simulink model "Sub_SC_G_based_221004"  (R2022b)
settings: Solver=VariableStepAuto  StartTime=0.0  StopTime=SimTime  RelTol=1e-3
undefined symbols (not defined in the file or in its folder): R_bal, SC_PreChgTime, SC_rc, SC_rv
libraries: spsCurrentMeasurementLib x14, spsSeriesRLCBranchLib x13, spsSupercapacitorLib x12, spsIdealSwitchLib x3, spsDCVoltageSourceLib x2, spsVariableResistorLib x2, spsVoltageMeasurementLib x1, sps_lib x1
settings Model: Creator=xuupp  LastModifiedBy=xuupp

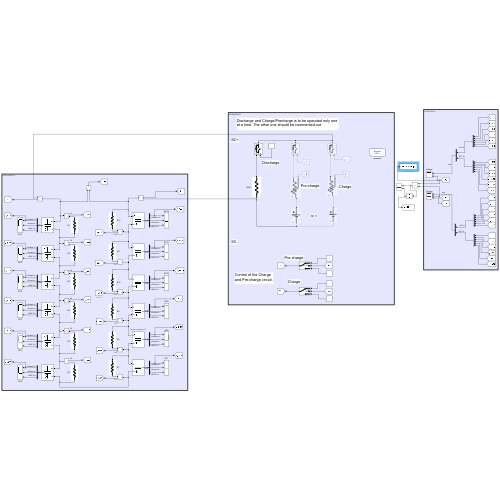
[thumbnail: Simulink's stored preview of the top-level diagram]
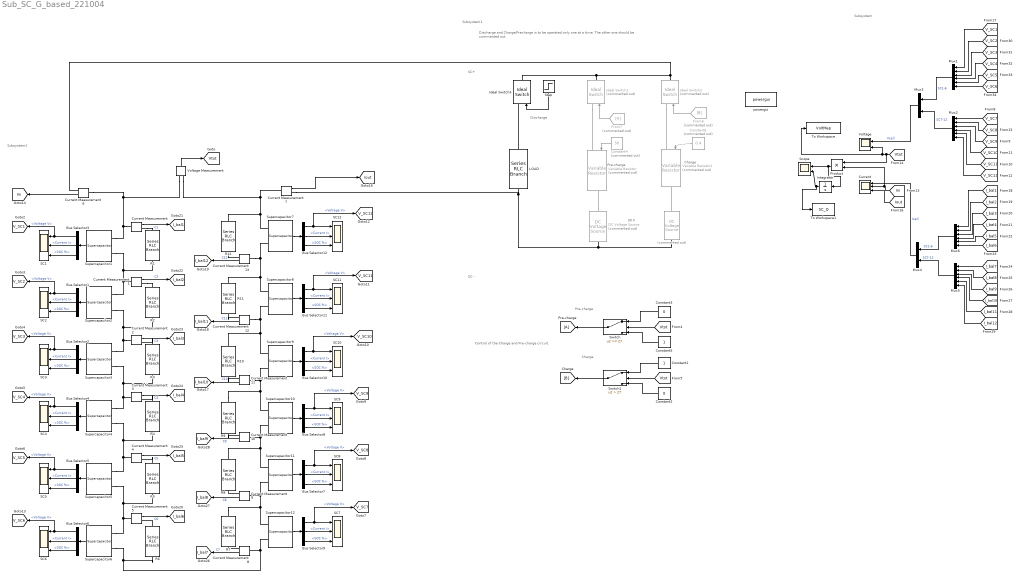
== system Sub_SC_G_based_221004 ==
  note: Pre-charge
  note: Subsystem2
  note: Control of the Charge and Pre-charge circuit.
  note: Subsystem
  note: 30 V
  note: Subsystem1
  note: SC -
  note: Charge
  note: Pre-charge
  note: SC+
  note: Discharge and Charge/Precharge is to be operated only one at a time. The other one should be commented out.
  note: Charge
  note: Discharge
  " " : spsDCVoltageSourceLib/DC Voltage Source  Commented=on  Amplitude=30  Measurements=None
  Bus Selector{1..12} (12 alike) : BusSelector  OutputSignals=Voltage V,Current I,SOC %
  Constant1 : Constant
  Constant2 : Constant  Value=0
  Constant3 : Constant  Value=0
  Constant4 : Constant  Commented=on  Value=30
  Constant5 : Constant
  Constant6 : Constant  Commented=on  Value=0.4
  Current : Scope  NumInputPorts=3
  Current Measurement{,1..13} (14 alike) : spsCurrentMeasurementLib/Current Measurement  PhasorSimulation=off  OutputType=Complex  PSBequivalent=0
  DC Voltage Source : spsDCVoltageSourceLib/DC Voltage Source  Commented=on  Amplitude=30  Measurements=None
  From6 : From  Commented=on  GotoTag=B
  From7 : From  Commented=on
  Ideal Switch1 : spsIdealSwitchLib/Ideal Switch  Commented=on  Ron=0.00001  Lon=0  IC=0  Rs=1e5  Cs=inf  Measurements=off
  Ideal Switch2 : spsIdealSwitchLib/Ideal Switch  Commented=on  Ron=0.00001  Lon=0  IC=0  Rs=1e5  Cs=inf  Measurements=off
  Ideal Switch3 : spsIdealSwitchLib/Ideal Switch  Ron=0.00001  Lon=0  IC=0  Rs=1e5  Cs=inf  Measurements=off
  Integrator : Integrator
  LOAD : spsSeriesRLCBranchLib/Series RLC Branch  LConnTagsString=__new0  RConnTagsString=__new0  BranchType=R  Resistance=10  Inductance=1e-3  SetiL0=off  InitialCurrent=0  Capacitance=1e-5  Setx0=on  InitialVoltage=0  Measurements=Branch voltage and current
  Mux{1..2,5..6} (4 alike) : Mux  Inputs=6
  Mux3 : Mux  Inputs=2
  Mux4 : Mux  Inputs=2
  Pre-charge : Goto
  Product : Product
  R{1..12} (12 alike) : spsSeriesRLCBranchLib/Series RLC Branch  LConnTagsString=__new0  RConnTagsString=__new0  BranchType=R  Resistance=R_bal  Inductance=1e-3  SetiL0=off  InitialCurrent=0  Capacitance=54.3e-6  Setx0=on  InitialVoltage=160  Measurements=None
  SC{1..12} (12 alike) : Scope  NumInputPorts=3
  Scope : Scope  NumInputPorts=2
  Step : Step  Time=SC_PreChgTime  SampleTime=0
  Supercapacitor{1..12} (12 alike) : spsSupercapacitorLib/Supercapacitor  C=SC_rc  Rdc=8.9e-3  Voltage=SC_rv  Ns=1  Np=1  Vinit=SC_iv  Temp=25  PresetModel=off  EstParam=off  Nc=1  r=1e-9  epsilon=6.0208e-10  Ich=10  Vstern="[0.161  2.7  7.8]"  Self_dis=on  Ioc=10  Vself="[48  47.8  47.06  44.65]"  demandeplot=off  I="[10  20 100  500]"  Units=sec  Vmax=0  If=0  deltaV=0  alpha=0  sec=0
      settings: LibrarySourceBlock=sps_lib/Sources/Supercapacitor
  Switch : Switch  Threshold=27  SaturateOnIntegerOverflow=off  InputSameDT=off
  Switch1 : Switch  Criteria=u2 > Threshold  Threshold=27  SaturateOnIntegerOverflow=off  InputSameDT=off
  To Workspace : ToWorkspace  VariableName=VoltMap  SaveFormat=Timeseries  SampleTime=-1
  To Workspace1 : ToWorkspace  VariableName=SC_Q  SaveFormat=Structure With Time  SampleTime=-1
  Variable Resistor : spsVariableResistorLib/Variable Resistor  Commented=on  Rabsmin=1e-3
      settings: LibrarySourceBlock=sps_lib/Passives/Variable Resistor
  Variable Resistor1 : spsVariableResistorLib/Variable Resistor  Commented=on  Rabsmin=1e-3
      settings: LibrarySourceBlock=sps_lib/Passives/Variable Resistor
  Voltage : Scope  NumInputPorts=2
  Voltage Measurement : spsVoltageMeasurementLib/Voltage Measurement  PhasorSimulation=off  OutputType=Complex  PSBequivalent=0
  powergui : sps_lib/powergui  Priority=1  SimulationMode=Discrete  SampleTime=0.01  frequency=60  Iterations=50  frequencyindice=0  Pbase=100e6  ErrMax=1e-4  UnitsV=kV  UnitsW=MW  buscounter=0  FunctionMessages=off  echomessages=off  EnableUseOfTLC=off  CurrentSourceSwitches=off  DisableSnubberDevices=off  DisableRonSwitches=off  DisableVfSwitches=off  DisplayEquations=off  AutomaticDiscreteSolvers=off  SolverType=Tustin/Backward Euler (TBE)  Interpol=off  ExternalGateDelay=off  methode=off  Ts=100  x0status=blocks  SPID=on  SwTol=0  HookPort=off  NonlinearTolerance=1e-4  nMaxIteration=100  ContinueOnMaxIteration=off  RestoreLinks=warning  ResistiveCurrentMeasurement=off  Frange=[0:2:500]  Ylog=off  Xlog=on  ShowGrid=off  save=off  variable=ZData  structure=0  ZoomFFT=off  StartTime=0.0  cycles=1  DisplayStyle=1  fundamental=60  FreqAxis=off  MaxFrequency=1000  frequencyindicesteady=1  RmsSteady=1  display=off
  tag scope: I_bal10=global, I_bal11=global, I_bal12=global, I_bal1=global, I_bal2=global, I_bal3=global, I_bal4=global, I_bal5=global, I_bal6=global, I_bal7=global, I_bal8=global, I_bal9=global, Iin=global, Iout=global, V_SC10=global, V_SC11=global, V_SC12=global, V_SC1=global, V_SC2=global, V_SC3=global, V_SC4=global, V_SC5=global, V_SC6=global, V_SC7=global, V_SC8=global, V_SC9=global, Vtot=global
  wires:
  Supercapacitor4/1 -> Bus Selector4/1
  Current Measurement12/1 -> [I_bal11]  "C11"
  Bus Selector12/3 -> SC12/3  "<SOC %>"
  [I_bal7] -> Mux5/1
  Bus Selector11/2 -> SC11/2  "<Current I>"
  Supercapacitor3/1 -> Bus Selector2/1
  Bus Selector2/3 -> SC3/3  "<SOC %>"
  Current Measurement11/1 -> [I_bal10]  "C10"
  Bus Selector1/2 -> SC2/2  "<Current I>"
  From7/1 -> Ideal Switch1/1
  Constant3/1 -> Switch/1
  Bus Selector3/1 -> [V_SC1], SC1/1  "<Voltage V>"
  Current Measurement8/1 -> [I_bal7]  "C7"
  Bus Selector1/3 -> SC2/3  "<SOC %>"
  Current Measurement1/1 -> [I_bal2]  "C2"
  Current Measurement5/1 -> [I_bal6]  "C6"
  Bus Selector5/1 -> [V_SC5], SC5/1  "<Voltage V>"
  Bus Selector10/2 -> SC10/2  "<Current I>"
  Bus Selector7/3 -> SC8/3  "<SOC %>"
  Bus Selector11/1 -> [V_SC11], SC11/1  "<Voltage V>"
  Bus Selector2/2 -> SC3/2  "<Current I>"
  Bus Selector4/3 -> SC4/3  "<SOC %>"
  Supercapacitor2/1 -> Bus Selector1/1
  Current Measurement/1 -> [I_bal1]  "C1"
  Bus Selector1/1 -> [V_SC2], SC2/1  "<Voltage V>"
  Bus Selector8/2 -> SC9/2  "<Current I>"
  Supercapacitor8/1 -> Bus Selector11/1
  Current Measurement2/1 -> [I_bal3]  "C3"
  Bus Selector8/3 -> SC9/3  "<SOC %>"
  Current Measurement6/1 -> [Iin]
  Bus Selector5/3 -> SC5/3  "<SOC %>"
  Bus Selector2/1 -> [V_SC3], SC3/1  "<Voltage V>"
  Bus Selector6/2 -> SC6/2  "<Current I>"
  Supercapacitor12/1 -> Bus Selector9/1
  Supercapacitor5/1 -> Bus Selector5/1
  Bus Selector12/2 -> SC12/2  "<Current I>"
  Supercapacitor7/1 -> Bus Selector12/1
  Bus Selector7/2 -> SC8/2  "<Current I>"
  Constant5/1 -> Switch/3
  Constant1/1 -> Switch1/1
  From6/1 -> Ideal Switch2/1
  [Vtot] -> Switch/2
  [Vtot] -> Switch1/2
  Switch/1 -> Pre-charge/1
  Step/1 -> Ideal Switch3/1
  Current Measurement9/1 -> [I_bal8]  "C8"
  Voltage Measurement/1 -> [Vtot]
  Current Measurement3/1 -> [I_bal4]  "C4"
  Constant4/1 -> Variable Resistor/1
  [V_SC4] -> Mux1/4
  [I_bal10] -> Mux5/4
  [V_SC12] -> Mux2/6
  [V_SC3] -> Mux1/3
  Bus Selector7/1 -> [V_SC8], SC8/1  "<Voltage V>"
  [I_bal3] -> Mux6/3
  [Vtot] -> Product/1, To Workspace/1, Voltage/2
  Bus Selector3/3 -> SC1/3  "<SOC %>"
  Supercapacitor6/1 -> Bus Selector6/1
  Bus Selector12/1 -> [V_SC12], SC12/1  "<Voltage V>"
  Bus Selector6/3 -> SC6/3  "<SOC %>"
  Bus Selector4/2 -> SC4/2  "<Current I>"
  Current Measurement10/1 -> [I_bal9]  "C9"
  Bus Selector6/1 -> [V_SC6], SC6/1  "<Voltage V>"
  [I_bal11] -> Mux5/5
  [V_SC8] -> Mux2/2
  [I_bal12] -> Mux5/6
  [I_bal2] -> Mux6/2
  [V_SC7] -> Mux2/1
  Constant6/1 -> Variable Resistor1/1
  Mux1/1 -> Mux3/1  "SC1-6"
  [I_bal9] -> Mux5/3
  Bus Selector10/3 -> SC10/3  "<SOC %>"
  Mux3/1 -> Voltage/1  "Vcell"
  [V_SC1] -> Mux1/1
  Bus Selector9/2 -> SC7/2  "<Current I>"
  Bus Selector9/1 -> [V_SC7], SC7/1  "<Voltage V>"
  Switch1/1 -> [B]
  Supercapacitor11/1 -> Bus Selector7/1
  [Iout] -> Current/3
  Bus Selector10/1 -> [V_SC10], SC10/1  "<Voltage V>"
  [V_SC9] -> Mux2/3
  Bus Selector11/3 -> SC11/3  "<SOC %>"
  Supercapacitor10/1 -> Bus Selector8/1
  Bus Selector9/3 -> SC7/3  "<SOC %>"
  Bus Selector8/1 -> [V_SC9], SC9/1  "<Voltage V>"
  [I_bal5] -> Mux6/5
  [I_bal8] -> Mux5/2
  Supercapacitor9/1 -> Bus Selector10/1
  [V_SC10] -> Mux2/4
  [I_bal4] -> Mux6/4
  Mux5/1 -> Mux4/2  "SC7-12"
  Bus Selector4/1 -> [V_SC4], SC4/1  "<Voltage V>"
  [V_SC2] -> Mux1/2
  Current Measurement7/1 -> [Iout]
  Bus Selector5/2 -> SC5/2  "<Current I>"
  Constant2/1 -> Switch1/3
  [V_SC5] -> Mux1/5
  [Iin] -> Product/2, Current/2
  Supercapacitor1/1 -> Bus Selector3/1
  Bus Selector3/2 -> SC1/2  "<Current I>"
  Current Measurement13/1 -> [I_bal12]  "C12"
  Mux4/1 -> Current/1  "Icell"
  Mux6/1 -> Mux4/1  "SC1-6"
  [I_bal1] -> Mux6/1
  [I_bal6] -> Mux6/6
  [V_SC11] -> Mux2/5
  Current Measurement4/1 -> [I_bal5]  "C5"
  [V_SC6] -> Mux1/6
  Mux2/1 -> Mux3/2  "SC7-12"
  Product/1 -> Integrator/1, Scope/1
  Integrator/1 -> To Workspace1/1, Scope/2
  connections:
  R6/RConn1 -- Supercapacitor6/LConn2 -- Supercapacitor12/LConn1 -- Current Measurement8/LConn1
  Current Measurement13/LConn1 -- Supercapacitor7/LConn1 -- Supercapacitor8/LConn2 -- R11/RConn1
  Current Measurement/LConn1 -- Supercapacitor1/LConn1 -- Voltage Measurement/LConn1 -- Current Measurement6/LConn1
  Current Measurement12/LConn1 -- Supercapacitor8/LConn1 -- Supercapacitor9/LConn2 -- R10/RConn1
  Current Measurement2/LConn1 -- Supercapacitor3/LConn1 -- Supercapacitor2/LConn2 -- R2/RConn1
  R9/RConn1 -- Supercapacitor10/LConn2 -- Supercapacitor9/LConn1 -- Current Measurement11/LConn1
  Current Measurement10/LConn1 -- Supercapacitor10/LConn1 -- Supercapacitor11/LConn2 -- R8/RConn1
  R1/RConn1 -- Supercapacitor1/LConn2 -- Supercapacitor2/LConn1 -- Current Measurement1/LConn1
  Ideal Switch3/RConn1 -- Ideal Switch1/RConn1 -- Ideal Switch2/RConn1 -- Current Measurement6/RConn1
  R4/RConn1 -- Supercapacitor4/LConn2 -- Supercapacitor5/LConn1 -- Current Measurement4/LConn1
  R5/RConn1 -- Supercapacitor5/LConn2 -- Supercapacitor6/LConn1 -- Current Measurement5/LConn1
  Voltage Measurement/LConn2 -- Supercapacitor7/LConn2 -- R12/RConn1 -- Current Measurement7/LConn1
  LOAD/RConn1 -- " "/LConn1 -- DC Voltage Source/LConn1 -- Current Measurement7/RConn1
  R7/RConn1 -- Supercapacitor12/LConn2 -- Supercapacitor11/LConn1 -- Current Measurement9/LConn1
  R3/RConn1 -- Supercapacitor3/LConn2 -- Supercapacitor4/LConn1 -- Current Measurement3/LConn1
  LOAD/LConn1 -- Ideal Switch3/LConn1
  R3/LConn1 -- Current Measurement2/RConn1
  " "/RConn1 -- Variable Resistor1/RConn1
  R12/LConn1 -- Current Measurement13/RConn1
  Ideal Switch1/LConn1 -- Variable Resistor/LConn1
  Current Measurement/RConn1 -- R1/LConn1
  R6/LConn1 -- Current Measurement5/RConn1
  Current Measurement1/RConn1 -- R2/LConn1
  Current Measurement8/RConn1 -- R7/LConn1
  R10/LConn1 -- Current Measurement11/RConn1
  DC Voltage Source/RConn1 -- Variable Resistor/RConn1
  Ideal Switch2/LConn1 -- Variable Resistor1/LConn1
  R9/LConn1 -- Current Measurement10/RConn1
  Current Measurement9/RConn1 -- R8/LConn1
  R5/LConn1 -- Current Measurement4/RConn1
  R11/LConn1 -- Current Measurement12/RConn1
  R4/LConn1 -- Current Measurement3/RConn1
